simulink model "warplab_mimo_4x4"  (Simulink 6.6)
settings: Solver=ode45  StartTime=0.0  StopTime=50000  RelTol=1e-3
undefined symbols (not defined in the file): gcbh, xlBlockLoadCallback, xlGetSimulinkPeriod
libraries: xbsIndex_r4 x305, WARP_Blockset x16
(part 3 of 4)

== system warplab_mimo_4x4/Posedge ==
  D : Inport
  Delay : xbsIndex_r4/Delay  en=off  latency=1  dbl_ovrd=off  reg_retiming=off  block_type=delay
      settings: infoedit=Hardware notes: A delay line is a chain, each link of which is an SRL16 followed by a flip-flop. If register retiming is enabled, the delay line is a chain of flip-flops.  block_version=8.2
  Inverter : xbsIndex_r4/Inverter  en=off  latency=0  dbl_ovrd=off  block_type=inv
      settings: block_version=8.2
  Logical : xbsIndex_r4/Logical  logical_function=AND  inputs=2  en=off  latency=0  precision=Full  arith_type=Unsigned  n_bits=16  bin_pt=0  align_bp=on  dbl_ovrd=off  block_type=logical
      settings: block_version=8.2
  Q : Outport
  wires:
  D/1 -> Inverter/1, Logical/1
  Inverter/1 -> Delay/1
  Delay/1 -> Logical/2
  Logical/1 -> Q/1

== system warplab_mimo_4x4/Posedge1 ==
  D : Inport
  Delay : xbsIndex_r4/Delay  en=off  latency=1  dbl_ovrd=off  reg_retiming=off  block_type=delay
      settings: infoedit=Hardware notes: A delay line is a chain, each link of which is an SRL16 followed by a flip-flop. If register retiming is enabled, the delay line is a chain of flip-flops.  block_version=8.2
  Inverter : xbsIndex_r4/Inverter  en=off  latency=0  dbl_ovrd=off  block_type=inv
      settings: block_version=8.2
  Logical : xbsIndex_r4/Logical  logical_function=AND  inputs=2  en=off  latency=0  precision=Full  arith_type=Unsigned  n_bits=16  bin_pt=0  align_bp=on  dbl_ovrd=off  block_type=logical
      settings: block_version=8.2
  Q : Outport
  wires:
  Logical/1 -> Q/1
  Delay/1 -> Logical/2
  Inverter/1 -> Delay/1
  D/1 -> Logical/1, Inverter/1

== system warplab_mimo_4x4/Posedge2 ==
  D : Inport
  Delay : xbsIndex_r4/Delay  en=off  latency=1  dbl_ovrd=off  reg_retiming=off  block_type=delay
      settings: infoedit=Hardware notes: A delay line is a chain, each link of which is an SRL16 followed by a flip-flop. If register retiming is enabled, the delay line is a chain of flip-flops.  block_version=8.2
  Inverter : xbsIndex_r4/Inverter  en=off  latency=0  dbl_ovrd=off  block_type=inv
      settings: block_version=8.2
  Logical : xbsIndex_r4/Logical  logical_function=AND  inputs=2  en=off  latency=0  precision=Full  arith_type=Unsigned  n_bits=16  bin_pt=0  align_bp=on  dbl_ovrd=off  block_type=logical
      settings: block_version=8.2
  Q : Outport
  wires:
  Logical/1 -> Q/1
  Delay/1 -> Logical/2
  Inverter/1 -> Delay/1
  D/1 -> Logical/1, Inverter/1

== system warplab_mimo_4x4/Radio 1 Rx Buffers ==
  I/Q : Inport
  Addr : Inport  Port=2
  WE : Inport  Port=3
  EN : Inport  Port=4
  Convert1 : xbsIndex_r4/Convert  arith_type=Boolean  n_bits=16  bin_pt=14  quantization=Truncate  overflow=Wrap  latency=0  dbl_ovrd=off  pipeline=off  block_type=convert
      settings: block_version=8.2
  Gateway Out : xbsIndex_r4/Gateway Out  hdl_port=off  timing_constraint=None  locs_specified=off  LOCs={}  block_type=gatewayout
      settings: infoedit="Gateway out block.  Converts Xilinx fixed point inputs into ouputs of type Simulink integer, double, or fixed point.<P><P>Hardware notes:  In hardware these blocks become top level output ports or are discarded, depending on how they are configured."  block_version=10.1.2
  Gateway Out1 : xbsIndex_r4/Gateway Out  hdl_port=off  timing_constraint=None  locs_specified=off  LOCs={}  block_type=gatewayout
      settings: infoedit="Gateway out block.  Converts Xilinx fixed point inputs into ouputs of type Simulink integer, double, or fixed point.<P><P>Hardware notes:  In hardware these blocks become top level output ports or are discarded, depending on how they are configured."  block_version=10.1.2
  Logical : xbsIndex_r4/Logical  logical_function=AND  inputs=2  en=off  latency=0  precision=Full  arith_type=Unsigned  n_bits=16  bin_pt=0  align_bp=on  dbl_ovrd=off  block_type=logical
      settings: block_version=9.1.01
  Radio 1 I/Q Buffer : Subsystem
  Scope : Scope  NumInputPorts=2
      settings: YMin=-5~-5  YMax=5~5  SaveName=ScopeData2  MaxDataPoints=40000
  wires:
  Logical/1 -> Gateway Out1/1, Radio 1 I/Q Buffer/3(WE)
  Addr/1 -> Gateway Out/1, Radio 1 I/Q Buffer/1(Addr_14b)
  WE/1 -> Logical/1
  EN/1 -> Convert1/1
  Convert1/1 -> Logical/2
  I/Q/1 -> Radio 1 I/Q Buffer/2(I/Q_32b)
  Gateway Out/1 -> Scope/1
  Gateway Out1/1 -> Scope/2

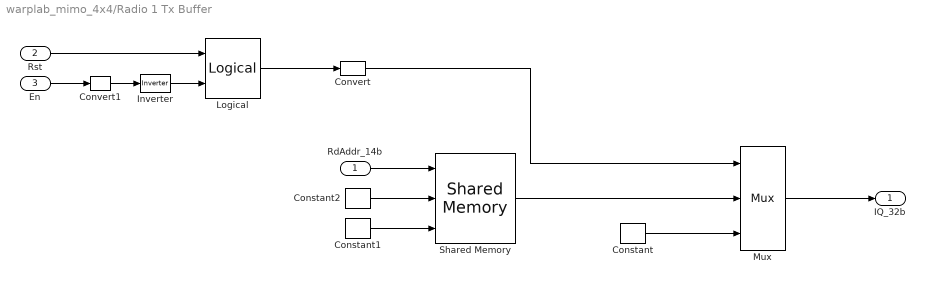
== system warplab_mimo_4x4/Radio 1 Tx Buffer ==
  RdAddr_14b : Inport
  Rst : Inport  Port=2
  En : Inport  Port=3
  Constant : xbsIndex_r4/Constant  arith_type=Unsigned  const=0  n_bits=32  bin_pt=0  explicit_period=off  period=1  equ=P=C  opselect=C  inp2=PCIN>>17  opr=+  inp1=P  carry=CIN  dbl_ovrd=off  block_type=constant
      settings: block_version=10.1.2
  Constant1 : xbsIndex_r4/Constant  arith_type=Boolean  const=0  n_bits=32  bin_pt=0  explicit_period=off  period=1  equ=P=C  opselect=C  inp2=PCIN>>17  opr=+  inp1=P  carry=CIN  dbl_ovrd=off  block_type=constant
      settings: block_version=10.1.2
  Constant2 : xbsIndex_r4/Constant  arith_type=Unsigned  const=0  n_bits=32  bin_pt=0  explicit_period=off  period=1  equ=P=C  opselect=C  inp2=PCIN>>17  opr=+  inp1=P  carry=CIN  dbl_ovrd=off  block_type=constant
      settings: block_version=10.1.2
  Convert : xbsIndex_r4/Convert  arith_type=Boolean  n_bits=16  bin_pt=14  quantization=Truncate  overflow=Wrap  latency=0  dbl_ovrd=off  pipeline=off  block_type=convert
      settings: block_version=8.2
  Convert1 : xbsIndex_r4/Convert  arith_type=Boolean  n_bits=16  bin_pt=14  quantization=Truncate  overflow=Wrap  latency=0  dbl_ovrd=off  pipeline=off  block_type=convert
      settings: block_version=8.2
  Inverter : xbsIndex_r4/Inverter  en=off  latency=0  dbl_ovrd=off  block_type=inv
      settings: block_version=9.1.01
  Logical : xbsIndex_r4/Logical  logical_function=OR  inputs=2  en=off  latency=0  precision=Full  arith_type=Unsigned  n_bits=16  bin_pt=0  align_bp=on  dbl_ovrd=off  block_type=logical
      settings: block_version=9.1.01
  Mux : xbsIndex_r4/Mux  inputs=2  en=off  latency=0  precision=Full  arith_type=Unsigned  n_bits=16  bin_pt=14  quantization=Truncate  overflow=Wrap  dbl_ovrd=off  block_type=mux
      settings: block_version=10.1.2
  Shared Memory : xbsIndex_r4/Shared Memory  shared_memory_name='TxBuff_Radio1'  depth=2^14  ownership=Locally Owned and Initialized  initVector=0  mutex=Unprotected  mode=Read and Write  write_mode=Read After Write  time_out=0  latency=1  explicit_data_type=on  arith_type=Unsigned  n_bits=32  bin_pt=0  implementation=Block RAM  use_rpm=off  block_type=shmem
      settings: AttributesFormatString=<< %<shared_memory_name> >>  block_version=10.1.2
  IQ_32b : Outport
  wires:
  Logical/1 -> Convert/1
  Convert/1 -> Mux/1
  Rst/1 -> Logical/1
  En/1 -> Convert1/1
  Convert1/1 -> Inverter/1
  Inverter/1 -> Logical/2
  RdAddr_14b/1 -> Shared Memory/1
  Constant/1 -> Mux/3
  Shared Memory/1 -> Mux/2
  Constant1/1 -> Shared Memory/3
  Constant2/1 -> Shared Memory/2
  Mux/1 -> IQ_32b/1

== system warplab_mimo_4x4/Radio 1 Inputs ==
  DebugRxBuffers : Inport
  ADC I : Subsystem
  ADC Q : Subsystem
  Concatenates_1 : Subsystem
  Gateway Out1 : xbsIndex_r4/Gateway Out  hdl_port=off  timing_constraint=None  locs_specified=off  LOCs={}  block_type=gatewayout
      settings: infoedit="Gateway out block.  Converts Xilinx fixed point inputs into ouputs of type Simulink integer, double, or fixed point.<P><P>Hardware notes:  In hardware these blocks become top level output ports or are discarded, depending on how they are configured."  block_version=10.1.2
  Gateway Out4 : xbsIndex_r4/Gateway Out  hdl_port=off  timing_constraint=None  locs_specified=off  LOCs={}  block_type=gatewayout
      settings: infoedit="Gateway out block.  Converts Xilinx fixed point inputs into ouputs of type Simulink integer, double, or fixed point.<P><P>Hardware notes:  In hardware these blocks become top level output ports or are discarded, depending on how they are configured."  block_version=10.1.2
  Scope : Scope  NumInputPorts=2
      settings: YMin=-5~-5  YMax=5~5
  Radio 1 I/Q : Outport
  wires:
  ADC Q/2(ADC Q) -> Concatenates_1/4(ADC_Q), Gateway Out1/1
  ADC Q/1(OTR Q) -> Concatenates_1/3(OTR_Q)
  ADC I/2(ADC I) -> Concatenates_1/2(ADC_I), Gateway Out4/1
  ADC I/1(OTR I) -> Concatenates_1/1(OTR_I)
  Concatenates_1/1(32b) -> Radio 1 I/Q/1
  Gateway Out4/1 -> Scope/1
  Gateway Out1/1 -> Scope/2
  DebugRxBuffers/1 -> ADC I/1(Debug), ADC Q/1(Debug)

== system warplab_mimo_4x4/Radio 1 Outputs ==
  32b : Inport
  16LSB : xbsIndex_r4/Slice  nbits=16  boolean_output=off  mode=Lower Bit Location + Width  bit1=0  base1=MSB of Input  bit0=0  base0=LSB of Input  dbl_ovrd=off  block_type=slice
      settings: infoedit="Extracts a given range of bits from each input sample and presents it at the output.  The output type is ordinarily unsigned with binary point at zero, but can be Boolean when the slice is one bit wide.<P><P>Hardware notes: In hardware this block costs nothing."  block_version=8.2
  16MSB : xbsIndex_r4/Slice  nbits=16  boolean_output=off  mode=Upper Bit Location + Width  bit1=0  base1=MSB of Input  bit0=0  base0=LSB of Input  dbl_ovrd=off  block_type=slice
      settings: infoedit="Extracts a given range of bits from each input sample and presents it at the output.  The output type is ordinarily unsigned with binary point at zero, but can be Boolean when the slice is one bit wide.<P><P>Hardware notes: In hardware this block costs nothing."  block_version=8.2
  Radio 1 DAC I : WARP_Blockset/WARP Radio Board ADC//DACs/Radio 1 DAC I  SystemSampleTime=-1
  Radio 1 DAC Q : WARP_Blockset/WARP Radio Board ADC//DACs/Radio 1 DAC Q  SystemSampleTime=-1
  Register : xbsIndex_r4/Register  init=0  rst=off  en=off  dbl_ovrd=off  block_type=register
      settings: block_version=8.2
  Register1 : xbsIndex_r4/Register  init=0  rst=off  en=off  dbl_ovrd=off  block_type=register
      settings: block_version=8.2
  Reinterpret : xbsIndex_r4/Reinterpret  force_arith_type=on  arith_type="Signed  (2's comp)"  force_bin_pt=on  bin_pt=15  block_type=reinterpret
      settings: infoedit="Changes signal type without altering the binary representation.   You can changed the signal between signed and unsigned, and relocate the binary point.<P><P>Hardware notes: In hardware this block costs nothing.<P><P>Example:  Suppose the input is 6 bits wide, signed, with 2 fractional bits, and the output is forced to unsigned with 0 fractional bits.  Then an input of -2.0 (1110.00 in binary 2's complement) becomes an output of 56 (111000 in binary)."  block_version=8.2
  Reinterpret1 : xbsIndex_r4/Reinterpret  force_arith_type=on  arith_type="Signed  (2's comp)"  force_bin_pt=on  bin_pt=15  block_type=reinterpret
      settings: infoedit="Changes signal type without altering the binary representation.   You can changed the signal between signed and unsigned, and relocate the binary point.<P><P>Hardware notes: In hardware this block costs nothing.<P><P>Example:  Suppose the input is 6 bits wide, signed, with 2 fractional bits, and the output is forced to unsigned with 0 fractional bits.  Then an input of -2.0 (1110.00 in binary 2's complement) becomes an output of 56 (111000 in binary)."  block_version=8.2
  Terminator1 : Terminator
  Terminator2 : Terminator
  wires:
  Radio 1 DAC Q/1 -> Terminator2/1
  Radio 1 DAC I/1 -> Terminator1/1
  Reinterpret1/1 -> Register1/1
  Reinterpret/1 -> Register/1
  16LSB/1 -> Reinterpret1/1
  16MSB/1 -> Reinterpret/1
  Register/1 -> Radio 1 DAC I/1
  Register1/1 -> Radio 1 DAC Q/1
  32b/1 -> 16MSB/1, 16LSB/1

== system warplab_mimo_4x4/Radio 2 Rx Buffers ==
  I/Q : Inport
  Addr : Inport  Port=2
  WE : Inport  Port=3
  EN : Inport  Port=4
  Convert1 : xbsIndex_r4/Convert  arith_type=Boolean  n_bits=16  bin_pt=14  quantization=Truncate  overflow=Wrap  latency=0  dbl_ovrd=off  pipeline=off  block_type=convert
      settings: block_version=8.2
  Gateway Out : xbsIndex_r4/Gateway Out  hdl_port=off  timing_constraint=None  locs_specified=off  LOCs={}  block_type=gatewayout
      settings: infoedit="Gateway out block.  Converts Xilinx fixed point inputs into ouputs of type Simulink integer, double, or fixed point.<P><P>Hardware notes:  In hardware these blocks become top level output ports or are discarded, depending on how they are configured."  block_version=10.1.2
  Gateway Out1 : xbsIndex_r4/Gateway Out  hdl_port=off  timing_constraint=None  locs_specified=off  LOCs={}  block_type=gatewayout
      settings: infoedit="Gateway out block.  Converts Xilinx fixed point inputs into ouputs of type Simulink integer, double, or fixed point.<P><P>Hardware notes:  In hardware these blocks become top level output ports or are discarded, depending on how they are configured."  block_version=10.1.2
  Logical : xbsIndex_r4/Logical  logical_function=AND  inputs=2  en=off  latency=0  precision=Full  arith_type=Unsigned  n_bits=16  bin_pt=0  align_bp=on  dbl_ovrd=off  block_type=logical
      settings: block_version=9.1.01
  Radio 2 I/Q Buffer : Subsystem
  Scope : Scope  NumInputPorts=2
      settings: YMin=-5~-5  YMax=5~5  SaveName=ScopeData2  MaxDataPoints=40000
  wires:
  Logical/1 -> Gateway Out1/1, Radio 2 I/Q Buffer/3(WE)
  Addr/1 -> Gateway Out/1, Radio 2 I/Q Buffer/1(Addr_14b)
  WE/1 -> Logical/1
  EN/1 -> Convert1/1
  Convert1/1 -> Logical/2
  I/Q/1 -> Radio 2 I/Q Buffer/2(I/Q_32b)
  Gateway Out/1 -> Scope/1
  Gateway Out1/1 -> Scope/2

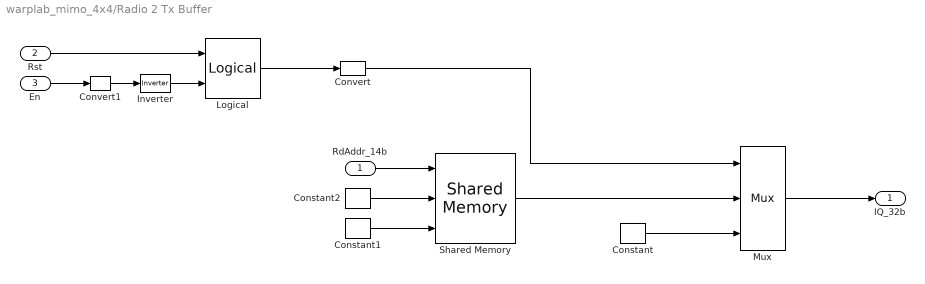
== system warplab_mimo_4x4/Radio 2 Tx Buffer ==
  RdAddr_14b : Inport
  Rst : Inport  Port=2
  En : Inport  Port=3
  Constant : xbsIndex_r4/Constant  arith_type=Unsigned  const=0  n_bits=32  bin_pt=0  explicit_period=off  period=1  equ=P=C  opselect=C  inp2=PCIN>>17  opr=+  inp1=P  carry=CIN  dbl_ovrd=off  block_type=constant
      settings: block_version=10.1.2
  Constant1 : xbsIndex_r4/Constant  arith_type=Boolean  const=0  n_bits=32  bin_pt=0  explicit_period=off  period=1  equ=P=C  opselect=C  inp2=PCIN>>17  opr=+  inp1=P  carry=CIN  dbl_ovrd=off  block_type=constant
      settings: block_version=10.1.2
  Constant2 : xbsIndex_r4/Constant  arith_type=Unsigned  const=0  n_bits=32  bin_pt=0  explicit_period=off  period=1  equ=P=C  opselect=C  inp2=PCIN>>17  opr=+  inp1=P  carry=CIN  dbl_ovrd=off  block_type=constant
      settings: block_version=10.1.2
  Convert : xbsIndex_r4/Convert  arith_type=Boolean  n_bits=16  bin_pt=14  quantization=Truncate  overflow=Wrap  latency=0  dbl_ovrd=off  pipeline=off  block_type=convert
      settings: block_version=8.2
  Convert1 : xbsIndex_r4/Convert  arith_type=Boolean  n_bits=16  bin_pt=14  quantization=Truncate  overflow=Wrap  latency=0  dbl_ovrd=off  pipeline=off  block_type=convert
      settings: block_version=8.2
  Inverter : xbsIndex_r4/Inverter  en=off  latency=0  dbl_ovrd=off  block_type=inv
      settings: block_version=9.1.01
  Logical : xbsIndex_r4/Logical  logical_function=OR  inputs=2  en=off  latency=0  precision=Full  arith_type=Unsigned  n_bits=16  bin_pt=0  align_bp=on  dbl_ovrd=off  block_type=logical
      settings: block_version=9.1.01
  Mux : xbsIndex_r4/Mux  inputs=2  en=off  latency=0  precision=Full  arith_type=Unsigned  n_bits=16  bin_pt=14  quantization=Truncate  overflow=Wrap  dbl_ovrd=off  block_type=mux
      settings: block_version=10.1.2
  Shared Memory : xbsIndex_r4/Shared Memory  shared_memory_name='TxBuff_Radio2'  depth=2^14  ownership=Locally Owned and Initialized  initVector=0  mutex=Unprotected  mode=Read and Write  write_mode=Read After Write  time_out=0  latency=1  explicit_data_type=on  arith_type=Unsigned  n_bits=32  bin_pt=0  implementation=Block RAM  use_rpm=off  block_type=shmem
      settings: AttributesFormatString=<< %<shared_memory_name> >>  block_version=10.1.2
  IQ_32b : Outport
  wires:
  Logical/1 -> Convert/1
  Convert/1 -> Mux/1
  Rst/1 -> Logical/1
  En/1 -> Convert1/1
  Convert1/1 -> Inverter/1
  Inverter/1 -> Logical/2
  RdAddr_14b/1 -> Shared Memory/1
  Constant/1 -> Mux/3
  Shared Memory/1 -> Mux/2
  Constant1/1 -> Shared Memory/3
  Constant2/1 -> Shared Memory/2
  Mux/1 -> IQ_32b/1

== system warplab_mimo_4x4/Radio 2 Inputs ==
  DebugRxBuffers : Inport
  ADC I : Subsystem
  ADC Q : Subsystem
  Concatenates_1 : Subsystem
  Gateway Out1 : xbsIndex_r4/Gateway Out  hdl_port=off  timing_constraint=None  locs_specified=off  LOCs={}  block_type=gatewayout
      settings: infoedit="Gateway out block.  Converts Xilinx fixed point inputs into ouputs of type Simulink integer, double, or fixed point.<P><P>Hardware notes:  In hardware these blocks become top level output ports or are discarded, depending on how they are configured."  block_version=10.1.2
  Gateway Out4 : xbsIndex_r4/Gateway Out  hdl_port=off  timing_constraint=None  locs_specified=off  LOCs={}  block_type=gatewayout
      settings: infoedit="Gateway out block.  Converts Xilinx fixed point inputs into ouputs of type Simulink integer, double, or fixed point.<P><P>Hardware notes:  In hardware these blocks become top level output ports or are discarded, depending on how they are configured."  block_version=10.1.2
  Scope : Scope  NumInputPorts=2
      settings: YMin=-5~-5  YMax=5~5
  Radio 2 I/Q : Outport
  wires:
  ADC Q/2(ADC Q) -> Concatenates_1/4(ADC_Q), Gateway Out1/1
  ADC Q/1(OTR Q) -> Concatenates_1/3(OTR_Q)
  ADC I/2(ADC I) -> Concatenates_1/2(ADC_I), Gateway Out4/1
  ADC I/1(OTR I) -> Concatenates_1/1(OTR_I)
  Concatenates_1/1(32b) -> Radio 2 I/Q/1
  Gateway Out4/1 -> Scope/1
  Gateway Out1/1 -> Scope/2
  DebugRxBuffers/1 -> ADC I/1(Debug), ADC Q/1(Debug)

== system warplab_mimo_4x4/Radio 2 Outputs ==
  32b : Inport
  16LSB : xbsIndex_r4/Slice  nbits=16  boolean_output=off  mode=Lower Bit Location + Width  bit1=0  base1=MSB of Input  bit0=0  base0=LSB of Input  dbl_ovrd=off  block_type=slice
      settings: infoedit="Extracts a given range of bits from each input sample and presents it at the output.  The output type is ordinarily unsigned with binary point at zero, but can be Boolean when the slice is one bit wide.<P><P>Hardware notes: In hardware this block costs nothing."  block_version=8.2
  16MSB : xbsIndex_r4/Slice  nbits=16  boolean_output=off  mode=Upper Bit Location + Width  bit1=0  base1=MSB of Input  bit0=0  base0=LSB of Input  dbl_ovrd=off  block_type=slice
      settings: infoedit="Extracts a given range of bits from each input sample and presents it at the output.  The output type is ordinarily unsigned with binary point at zero, but can be Boolean when the slice is one bit wide.<P><P>Hardware notes: In hardware this block costs nothing."  block_version=8.2
  Radio 2 DAC I : WARP_Blockset/WARP Radio Board ADC//DACs/Radio 2 DAC I  SystemSampleTime=-1
  Radio 2 DAC Q : WARP_Blockset/WARP Radio Board ADC//DACs/Radio 2 DAC Q  SystemSampleTime=-1
  Register : xbsIndex_r4/Register  init=0  rst=off  en=off  dbl_ovrd=off  block_type=register
      settings: block_version=8.2
  Register1 : xbsIndex_r4/Register  init=0  rst=off  en=off  dbl_ovrd=off  block_type=register
      settings: block_version=8.2
  Reinterpret : xbsIndex_r4/Reinterpret  force_arith_type=on  arith_type="Signed  (2's comp)"  force_bin_pt=on  bin_pt=15  block_type=reinterpret
      settings: infoedit="Changes signal type without altering the binary representation.   You can changed the signal between signed and unsigned, and relocate the binary point.<P><P>Hardware notes: In hardware this block costs nothing.<P><P>Example:  Suppose the input is 6 bits wide, signed, with 2 fractional bits, and the output is forced to unsigned with 0 fractional bits.  Then an input of -2.0 (1110.00 in binary 2's complement) becomes an output of 56 (111000 in binary)."  block_version=8.2
  Reinterpret1 : xbsIndex_r4/Reinterpret  force_arith_type=on  arith_type="Signed  (2's comp)"  force_bin_pt=on  bin_pt=15  block_type=reinterpret
      settings: infoedit="Changes signal type without altering the binary representation.   You can changed the signal between signed and unsigned, and relocate the binary point.<P><P>Hardware notes: In hardware this block costs nothing.<P><P>Example:  Suppose the input is 6 bits wide, signed, with 2 fractional bits, and the output is forced to unsigned with 0 fractional bits.  Then an input of -2.0 (1110.00 in binary 2's complement) becomes an output of 56 (111000 in binary)."  block_version=8.2
  Terminator1 : Terminator
  Terminator2 : Terminator
  wires:
  Radio 2 DAC Q/1 -> Terminator2/1
  Radio 2 DAC I/1 -> Terminator1/1
  Reinterpret1/1 -> Register1/1
  Reinterpret/1 -> Register/1
  16LSB/1 -> Reinterpret1/1
  16MSB/1 -> Reinterpret/1
  Register/1 -> Radio 2 DAC I/1
  Register1/1 -> Radio 2 DAC Q/1
  32b/1 -> 16MSB/1, 16LSB/1

== system warplab_mimo_4x4/Radio 3 Rx Buffers ==
  I/Q : Inport
  Addr : Inport  Port=2
  WE : Inport  Port=3
  EN : Inport  Port=4
  Convert1 : xbsIndex_r4/Convert  arith_type=Boolean  n_bits=16  bin_pt=14  quantization=Truncate  overflow=Wrap  latency=0  dbl_ovrd=off  pipeline=off  block_type=convert
      settings: block_version=8.2
  Gateway Out : xbsIndex_r4/Gateway Out  hdl_port=off  timing_constraint=None  locs_specified=off  LOCs={}  block_type=gatewayout
      settings: infoedit="Gateway out block.  Converts Xilinx fixed point inputs into ouputs of type Simulink integer, double, or fixed point.<P><P>Hardware notes:  In hardware these blocks become top level output ports or are discarded, depending on how they are configured."  block_version=10.1.2
  Gateway Out1 : xbsIndex_r4/Gateway Out  hdl_port=off  timing_constraint=None  locs_specified=off  LOCs={}  block_type=gatewayout
      settings: infoedit="Gateway out block.  Converts Xilinx fixed point inputs into ouputs of type Simulink integer, double, or fixed point.<P><P>Hardware notes:  In hardware these blocks become top level output ports or are discarded, depending on how they are configured."  block_version=10.1.2
  Logical : xbsIndex_r4/Logical  logical_function=AND  inputs=2  en=off  latency=0  precision=Full  arith_type=Unsigned  n_bits=16  bin_pt=0  align_bp=on  dbl_ovrd=off  block_type=logical
      settings: block_version=9.1.01
  Radio 3 I/Q Buffer : Subsystem
  Scope : Scope  NumInputPorts=2
      settings: YMin=-5~-5  YMax=5~5  SaveName=ScopeData2  MaxDataPoints=40000
  wires:
  Gateway Out1/1 -> Scope/2
  Gateway Out/1 -> Scope/1
  I/Q/1 -> Radio 3 I/Q Buffer/2(I/Q_32b)
  Convert1/1 -> Logical/2
  EN/1 -> Convert1/1
  WE/1 -> Logical/1
  Addr/1 -> Gateway Out/1, Radio 3 I/Q Buffer/1(Addr_14b)
  Logical/1 -> Gateway Out1/1, Radio 3 I/Q Buffer/3(WE)

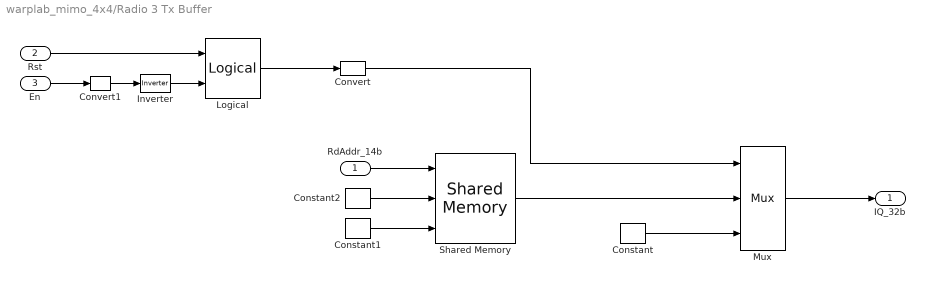
== system warplab_mimo_4x4/Radio 3 Tx Buffer ==
  RdAddr_14b : Inport
  Rst : Inport  Port=2
  En : Inport  Port=3
  Constant : xbsIndex_r4/Constant  arith_type=Unsigned  const=0  n_bits=32  bin_pt=0  explicit_period=off  period=1  equ=P=C  opselect=C  inp2=PCIN>>17  opr=+  inp1=P  carry=CIN  dbl_ovrd=off  block_type=constant
      settings: block_version=10.1.2
  Constant1 : xbsIndex_r4/Constant  arith_type=Boolean  const=0  n_bits=32  bin_pt=0  explicit_period=off  period=1  equ=P=C  opselect=C  inp2=PCIN>>17  opr=+  inp1=P  carry=CIN  dbl_ovrd=off  block_type=constant
      settings: block_version=10.1.2
  Constant2 : xbsIndex_r4/Constant  arith_type=Unsigned  const=0  n_bits=32  bin_pt=0  explicit_period=off  period=1  equ=P=C  opselect=C  inp2=PCIN>>17  opr=+  inp1=P  carry=CIN  dbl_ovrd=off  block_type=constant
      settings: block_version=10.1.2
  Convert : xbsIndex_r4/Convert  arith_type=Boolean  n_bits=16  bin_pt=14  quantization=Truncate  overflow=Wrap  latency=0  dbl_ovrd=off  pipeline=off  block_type=convert
      settings: block_version=8.2
  Convert1 : xbsIndex_r4/Convert  arith_type=Boolean  n_bits=16  bin_pt=14  quantization=Truncate  overflow=Wrap  latency=0  dbl_ovrd=off  pipeline=off  block_type=convert
      settings: block_version=8.2
  Inverter : xbsIndex_r4/Inverter  en=off  latency=0  dbl_ovrd=off  block_type=inv
      settings: block_version=9.1.01
  Logical : xbsIndex_r4/Logical  logical_function=OR  inputs=2  en=off  latency=0  precision=Full  arith_type=Unsigned  n_bits=16  bin_pt=0  align_bp=on  dbl_ovrd=off  block_type=logical
      settings: block_version=9.1.01
  Mux : xbsIndex_r4/Mux  inputs=2  en=off  latency=0  precision=Full  arith_type=Unsigned  n_bits=16  bin_pt=14  quantization=Truncate  overflow=Wrap  dbl_ovrd=off  block_type=mux
      settings: block_version=10.1.2
  Shared Memory : xbsIndex_r4/Shared Memory  shared_memory_name='TxBuff_Radio3'  depth=2^14  ownership=Locally Owned and Initialized  initVector=0  mutex=Unprotected  mode=Read and Write  write_mode=Read After Write  time_out=0  latency=1  explicit_data_type=on  arith_type=Unsigned  n_bits=32  bin_pt=0  implementation=Block RAM  use_rpm=off  block_type=shmem
      settings: AttributesFormatString=<< %<shared_memory_name> >>  block_version=10.1.2
  IQ_32b : Outport
  wires:
  Mux/1 -> IQ_32b/1
  Constant2/1 -> Shared Memory/2
  Constant1/1 -> Shared Memory/3
  Shared Memory/1 -> Mux/2
  Constant/1 -> Mux/3
  RdAddr_14b/1 -> Shared Memory/1
  Inverter/1 -> Logical/2
  Convert1/1 -> Inverter/1
  En/1 -> Convert1/1
  Rst/1 -> Logical/1
  Convert/1 -> Mux/1
  Logical/1 -> Convert/1

== system warplab_mimo_4x4/Radio 3 Inputs ==
  DebugRxBuffers : Inport
  ADC I : Subsystem
  ADC Q : Subsystem
  Concatenates_1 : Subsystem
  Gateway Out1 : xbsIndex_r4/Gateway Out  hdl_port=off  timing_constraint=None  locs_specified=off  LOCs={}  block_type=gatewayout
      settings: infoedit="Gateway out block.  Converts Xilinx fixed point inputs into ouputs of type Simulink integer, double, or fixed point.<P><P>Hardware notes:  In hardware these blocks become top level output ports or are discarded, depending on how they are configured."  block_version=10.1.2
  Gateway Out4 : xbsIndex_r4/Gateway Out  hdl_port=off  timing_constraint=None  locs_specified=off  LOCs={}  block_type=gatewayout
      settings: infoedit="Gateway out block.  Converts Xilinx fixed point inputs into ouputs of type Simulink integer, double, or fixed point.<P><P>Hardware notes:  In hardware these blocks become top level output ports or are discarded, depending on how they are configured."  block_version=10.1.2
  Scope : Scope  NumInputPorts=2
      settings: YMin=-5~-5  YMax=5~5
  Radio 3 I/Q : Outport
  wires:
  ADC Q/2(ADC Q) -> Concatenates_1/4(ADC_Q), Gateway Out1/1
  ADC Q/1(OTR Q) -> Concatenates_1/3(OTR_Q)
  ADC I/2(ADC I) -> Concatenates_1/2(ADC_I), Gateway Out4/1
  ADC I/1(OTR I) -> Concatenates_1/1(OTR_I)
  Concatenates_1/1(32b) -> Radio 3 I/Q/1
  Gateway Out4/1 -> Scope/1
  Gateway Out1/1 -> Scope/2
  DebugRxBuffers/1 -> ADC I/1(Debug), ADC Q/1(Debug)

== system warplab_mimo_4x4/Radio 3 Outputs ==
  32b : Inport
  16LSB : xbsIndex_r4/Slice  nbits=16  boolean_output=off  mode=Lower Bit Location + Width  bit1=0  base1=MSB of Input  bit0=0  base0=LSB of Input  dbl_ovrd=off  block_type=slice
      settings: infoedit="Extracts a given range of bits from each input sample and presents it at the output.  The output type is ordinarily unsigned with binary point at zero, but can be Boolean when the slice is one bit wide.<P><P>Hardware notes: In hardware this block costs nothing."  block_version=9.1.01
  16MSB : xbsIndex_r4/Slice  nbits=16  boolean_output=off  mode=Upper Bit Location + Width  bit1=0  base1=MSB of Input  bit0=0  base0=LSB of Input  dbl_ovrd=off  block_type=slice
      settings: infoedit="Extracts a given range of bits from each input sample and presents it at the output.  The output type is ordinarily unsigned with binary point at zero, but can be Boolean when the slice is one bit wide.<P><P>Hardware notes: In hardware this block costs nothing."  block_version=9.1.01
  Radio 3 DAC I : WARP_Blockset/WARP Radio Board ADC//DACs/Radio 3 DAC I  SystemSampleTime=-1
  Radio 3 DAC Q : WARP_Blockset/WARP Radio Board ADC//DACs/Radio 3 DAC Q  SystemSampleTime=-1
  Register : xbsIndex_r4/Register  init=0  rst=off  en=off  dbl_ovrd=off  block_type=register
      settings: block_version=9.1.01
  Register1 : xbsIndex_r4/Register  init=0  rst=off  en=off  dbl_ovrd=off  block_type=register
      settings: block_version=9.1.01
  Reinterpret : xbsIndex_r4/Reinterpret  force_arith_type=on  arith_type="Signed  (2's comp)"  force_bin_pt=on  bin_pt=15  block_type=reinterpret
      settings: infoedit="Changes signal type without altering the binary representation.   You can changed the signal between signed and unsigned, and relocate the binary point.<P><P>Hardware notes: In hardware this block costs nothing.<P><P>Example:  Suppose the input is 6 bits wide, signed, with 2 fractional bits, and the output is forced to unsigned with 0 fractional bits.  Then an input of -2.0 (1110.00 in binary 2's complement) becomes an output of 56 (111000 in binary)."  block_version=9.1.01
  Reinterpret1 : xbsIndex_r4/Reinterpret  force_arith_type=on  arith_type="Signed  (2's comp)"  force_bin_pt=on  bin_pt=15  block_type=reinterpret
      settings: infoedit="Changes signal type without altering the binary representation.   You can changed the signal between signed and unsigned, and relocate the binary point.<P><P>Hardware notes: In hardware this block costs nothing.<P><P>Example:  Suppose the input is 6 bits wide, signed, with 2 fractional bits, and the output is forced to unsigned with 0 fractional bits.  Then an input of -2.0 (1110.00 in binary 2's complement) becomes an output of 56 (111000 in binary)."  block_version=9.1.01
  Terminator : Terminator
  Terminator1 : Terminator
  wires:
  32b/1 -> 16LSB/1, 16MSB/1
  16MSB/1 -> Reinterpret/1
  16LSB/1 -> Reinterpret1/1
  Reinterpret/1 -> Register/1
  Reinterpret1/1 -> Register1/1
  Register/1 -> Radio 3 DAC I/1
  Register1/1 -> Radio 3 DAC Q/1
  Radio 3 DAC I/1 -> Terminator/1
  Radio 3 DAC Q/1 -> Terminator1/1

== system warplab_mimo_4x4/Radio 4 Rx Buffers ==
  I/Q : Inport
  Addr : Inport  Port=2
  WE : Inport  Port=3
  EN : Inport  Port=4
  Convert1 : xbsIndex_r4/Convert  arith_type=Boolean  n_bits=16  bin_pt=14  quantization=Truncate  overflow=Wrap  latency=0  dbl_ovrd=off  pipeline=off  block_type=convert
      settings: block_version=8.2
  Gateway Out : xbsIndex_r4/Gateway Out  hdl_port=off  timing_constraint=None  locs_specified=off  LOCs={}  block_type=gatewayout
      settings: infoedit="Gateway out block.  Converts Xilinx fixed point inputs into ouputs of type Simulink integer, double, or fixed point.<P><P>Hardware notes:  In hardware these blocks become top level output ports or are discarded, depending on how they are configured."  block_version=10.1.2
  Gateway Out1 : xbsIndex_r4/Gateway Out  hdl_port=off  timing_constraint=None  locs_specified=off  LOCs={}  block_type=gatewayout
      settings: infoedit="Gateway out block.  Converts Xilinx fixed point inputs into ouputs of type Simulink integer, double, or fixed point.<P><P>Hardware notes:  In hardware these blocks become top level output ports or are discarded, depending on how they are configured."  block_version=10.1.2
  Logical : xbsIndex_r4/Logical  logical_function=AND  inputs=2  en=off  latency=0  precision=Full  arith_type=Unsigned  n_bits=16  bin_pt=0  align_bp=on  dbl_ovrd=off  block_type=logical
      settings: block_version=9.1.01
  Radio 4 I/Q Buffer : Subsystem
  Scope : Scope  NumInputPorts=2
      settings: YMin=-5~-5  YMax=5~5  SaveName=ScopeData2  MaxDataPoints=40000
  wires:
  Gateway Out1/1 -> Scope/2
  Gateway Out/1 -> Scope/1
  I/Q/1 -> Radio 4 I/Q Buffer/2(I/Q_32b)
  Convert1/1 -> Logical/2
  EN/1 -> Convert1/1
  WE/1 -> Logical/1
  Addr/1 -> Gateway Out/1, Radio 4 I/Q Buffer/1(Addr_14b)
  Logical/1 -> Gateway Out1/1, Radio 4 I/Q Buffer/3(WE)

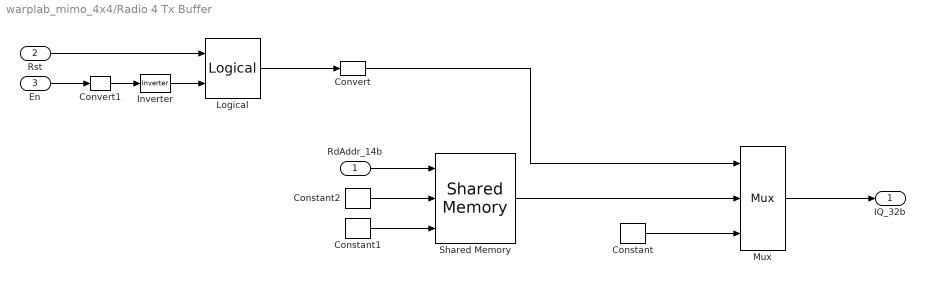
== system warplab_mimo_4x4/Radio 4 Tx Buffer ==
  RdAddr_14b : Inport
  Rst : Inport  Port=2
  En : Inport  Port=3
  Constant : xbsIndex_r4/Constant  arith_type=Unsigned  const=0  n_bits=32  bin_pt=0  explicit_period=off  period=1  equ=P=C  opselect=C  inp2=PCIN>>17  opr=+  inp1=P  carry=CIN  dbl_ovrd=off  block_type=constant
      settings: block_version=10.1.2
  Constant1 : xbsIndex_r4/Constant  arith_type=Boolean  const=0  n_bits=32  bin_pt=0  explicit_period=off  period=1  equ=P=C  opselect=C  inp2=PCIN>>17  opr=+  inp1=P  carry=CIN  dbl_ovrd=off  block_type=constant
      settings: block_version=10.1.2
  Constant2 : xbsIndex_r4/Constant  arith_type=Unsigned  const=0  n_bits=32  bin_pt=0  explicit_period=off  period=1  equ=P=C  opselect=C  inp2=PCIN>>17  opr=+  inp1=P  carry=CIN  dbl_ovrd=off  block_type=constant
      settings: block_version=10.1.2
  Convert : xbsIndex_r4/Convert  arith_type=Boolean  n_bits=16  bin_pt=14  quantization=Truncate  overflow=Wrap  latency=0  dbl_ovrd=off  pipeline=off  block_type=convert
      settings: block_version=8.2
  Convert1 : xbsIndex_r4/Convert  arith_type=Boolean  n_bits=16  bin_pt=14  quantization=Truncate  overflow=Wrap  latency=0  dbl_ovrd=off  pipeline=off  block_type=convert
      settings: block_version=8.2
  Inverter : xbsIndex_r4/Inverter  en=off  latency=0  dbl_ovrd=off  block_type=inv
      settings: block_version=9.1.01
  Logical : xbsIndex_r4/Logical  logical_function=OR  inputs=2  en=off  latency=0  precision=Full  arith_type=Unsigned  n_bits=16  bin_pt=0  align_bp=on  dbl_ovrd=off  block_type=logical
      settings: block_version=9.1.01
  Mux : xbsIndex_r4/Mux  inputs=2  en=off  latency=0  precision=Full  arith_type=Unsigned  n_bits=16  bin_pt=14  quantization=Truncate  overflow=Wrap  dbl_ovrd=off  block_type=mux
      settings: block_version=10.1.2
  Shared Memory : xbsIndex_r4/Shared Memory  shared_memory_name='TxBuff_Radio4'  depth=2^14  ownership=Locally Owned and Initialized  initVector=0  mutex=Unprotected  mode=Read and Write  write_mode=Read After Write  time_out=0  latency=1  explicit_data_type=on  arith_type=Unsigned  n_bits=32  bin_pt=0  implementation=Block RAM  use_rpm=off  block_type=shmem
      settings: AttributesFormatString=<< %<shared_memory_name> >>  block_version=10.1.2
  IQ_32b : Outport
  wires:
  Mux/1 -> IQ_32b/1
  Constant2/1 -> Shared Memory/2
  Constant1/1 -> Shared Memory/3
  Shared Memory/1 -> Mux/2
  Constant/1 -> Mux/3
  RdAddr_14b/1 -> Shared Memory/1
  Inverter/1 -> Logical/2
  Convert1/1 -> Inverter/1
  En/1 -> Convert1/1
  Rst/1 -> Logical/1
  Convert/1 -> Mux/1
  Logical/1 -> Convert/1

== system warplab_mimo_4x4/Radio 4 Inputs ==
  DebugRxBuffers : Inport
  ADC I : Subsystem
  ADC Q : Subsystem
  Concatenates_1 : Subsystem
  Gateway Out1 : xbsIndex_r4/Gateway Out  hdl_port=off  timing_constraint=None  locs_specified=off  LOCs={}  block_type=gatewayout
      settings: infoedit="Gateway out block.  Converts Xilinx fixed point inputs into ouputs of type Simulink integer, double, or fixed point.<P><P>Hardware notes:  In hardware these blocks become top level output ports or are discarded, depending on how they are configured."  block_version=10.1.2
  Gateway Out4 : xbsIndex_r4/Gateway Out  hdl_port=off  timing_constraint=None  locs_specified=off  LOCs={}  block_type=gatewayout
      settings: infoedit="Gateway out block.  Converts Xilinx fixed point inputs into ouputs of type Simulink integer, double, or fixed point.<P><P>Hardware notes:  In hardware these blocks become top level output ports or are discarded, depending on how they are configured."  block_version=10.1.2
  Scope : Scope  NumInputPorts=2
      settings: YMin=-5~-5  YMax=5~5
  Radio 4 I/Q : Outport
  wires:
  ADC Q/2(ADC Q) -> Concatenates_1/4(ADC_Q), Gateway Out1/1
  ADC Q/1(OTR Q) -> Concatenates_1/3(OTR_Q)
  ADC I/2(ADC I) -> Concatenates_1/2(ADC_I), Gateway Out4/1
  ADC I/1(OTR I) -> Concatenates_1/1(OTR_I)
  Concatenates_1/1(32b) -> Radio 4 I/Q/1
  Gateway Out4/1 -> Scope/1
  Gateway Out1/1 -> Scope/2
  DebugRxBuffers/1 -> ADC I/1(Debug), ADC Q/1(Debug)

== system warplab_mimo_4x4/Radio 4 Outputs ==
  32b : Inport
  16LSB : xbsIndex_r4/Slice  nbits=16  boolean_output=off  mode=Lower Bit Location + Width  bit1=0  base1=MSB of Input  bit0=0  base0=LSB of Input  dbl_ovrd=off  block_type=slice
      settings: infoedit="Extracts a given range of bits from each input sample and presents it at the output.  The output type is ordinarily unsigned with binary point at zero, but can be Boolean when the slice is one bit wide.<P><P>Hardware notes: In hardware this block costs nothing."  block_version=9.1.01
  16MSB : xbsIndex_r4/Slice  nbits=16  boolean_output=off  mode=Upper Bit Location + Width  bit1=0  base1=MSB of Input  bit0=0  base0=LSB of Input  dbl_ovrd=off  block_type=slice
      settings: infoedit="Extracts a given range of bits from each input sample and presents it at the output.  The output type is ordinarily unsigned with binary point at zero, but can be Boolean when the slice is one bit wide.<P><P>Hardware notes: In hardware this block costs nothing."  block_version=9.1.01
  Radio 4 DAC I : WARP_Blockset/WARP Radio Board ADC//DACs/Radio 4 DAC I  SystemSampleTime=-1
  Radio 4 DAC Q : WARP_Blockset/WARP Radio Board ADC//DACs/Radio 4 DAC Q  SystemSampleTime=-1
  Register : xbsIndex_r4/Register  init=0  rst=off  en=off  dbl_ovrd=off  block_type=register
      settings: block_version=9.1.01
  Register1 : xbsIndex_r4/Register  init=0  rst=off  en=off  dbl_ovrd=off  block_type=register
      settings: block_version=9.1.01
  Reinterpret : xbsIndex_r4/Reinterpret  force_arith_type=on  arith_type="Signed  (2's comp)"  force_bin_pt=on  bin_pt=15  block_type=reinterpret
      settings: infoedit="Changes signal type without altering the binary representation.   You can changed the signal between signed and unsigned, and relocate the binary point.<P><P>Hardware notes: In hardware this block costs nothing.<P><P>Example:  Suppose the input is 6 bits wide, signed, with 2 fractional bits, and the output is forced to unsigned with 0 fractional bits.  Then an input of -2.0 (1110.00 in binary 2's complement) becomes an output of 56 (111000 in binary)."  block_version=9.1.01
  Reinterpret1 : xbsIndex_r4/Reinterpret  force_arith_type=on  arith_type="Signed  (2's comp)"  force_bin_pt=on  bin_pt=15  block_type=reinterpret
      settings: infoedit="Changes signal type without altering the binary representation.   You can changed the signal between signed and unsigned, and relocate the binary point.<P><P>Hardware notes: In hardware this block costs nothing.<P><P>Example:  Suppose the input is 6 bits wide, signed, with 2 fractional bits, and the output is forced to unsigned with 0 fractional bits.  Then an input of -2.0 (1110.00 in binary 2's complement) becomes an output of 56 (111000 in binary)."  block_version=9.1.01
  Terminator : Terminator
  Terminator1 : Terminator
  wires:
  32b/1 -> 16LSB/1, 16MSB/1
  16MSB/1 -> Reinterpret/1
  16LSB/1 -> Reinterpret1/1
  Reinterpret/1 -> Register/1
  Reinterpret1/1 -> Register1/1
  Register/1 -> Radio 4 DAC I/1
  Register1/1 -> Radio 4 DAC Q/1
  Radio 4 DAC I/1 -> Terminator/1
  Radio 4 DAC Q/1 -> Terminator1/1

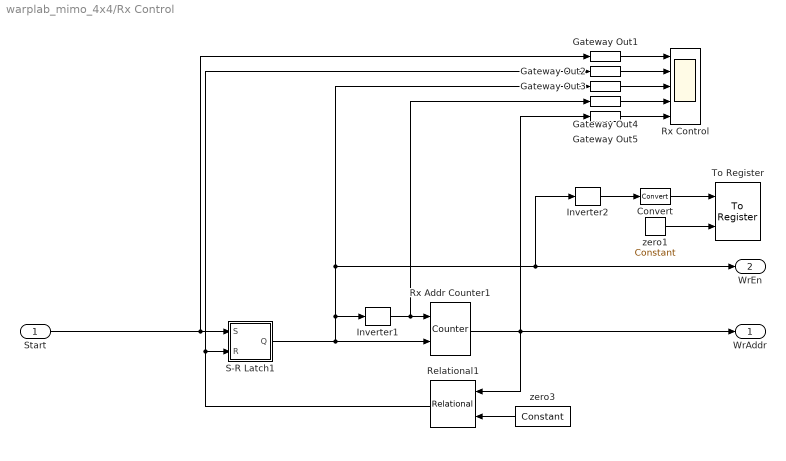
== system warplab_mimo_4x4/Rx Control ==
  Start : Inport
  Convert : xbsIndex_r4/Convert  arith_type=Unsigned  n_bits=1  bin_pt=0  quantization=Truncate  overflow=Wrap  latency=0  dbl_ovrd=off  pipeline=off  block_type=convert
      settings: block_version=10.1.2
  Gateway Out{1..5} (5 alike) : xbsIndex_r4/Gateway Out  hdl_port=off  timing_constraint=None  locs_specified=off  LOCs={}  block_type=gatewayout
      settings: infoedit="Gateway out block.  Converts Xilinx fixed point inputs into ouputs of type Simulink integer, double, or fixed point.<P><P>Hardware notes:  In hardware these blocks become top level output ports or are discarded, depending on how they are configured."  block_version=10.1.2
  Inverter1 : xbsIndex_r4/Inverter  en=off  latency=0  dbl_ovrd=off  block_type=inv
      settings: block_version=8.2
  Inverter2 : xbsIndex_r4/Inverter  en=off  latency=0  dbl_ovrd=off  block_type=inv
      settings: block_version=8.2
  Relational1 : xbsIndex_r4/Relational  Orientation=left  mode=a>=b  en=off  latency=0  dbl_ovrd=off  block_type=relational
      settings: block_version=8.2
  Rx Addr Counter1 : xbsIndex_r4/Counter  cnt_type=Free Running  cnt_to=Inf  operation=Up  start_count=0  cnt_by_val=1  arith_type=Unsigned  n_bits=14  bin_pt=0  load_pin=off  rst=on  en=on  explicit_period=off  period=1  dbl_ovrd=off  use_behavioral_HDL=off  use_rpm=off  implementation=Fabric  block_type=counter
      settings: block_version=8.2
  Rx Control : Scope  NumInputPorts=5
      settings: TimeRange=70000  YMin=0~0~0~0~0  YMax=1~1~1~1~20000
  S-R Latch1 : Subsystem
  To Register : xbsIndex_r4/To Register  shared_memory_name='CaptureDone'  init=0  ownership=Locally owned and initialized  explicit_data_type=on  arith_type=Unsigned  n_bits=1  bin_pt=0  dbl_ovrd=off  block_type=toreg
      settings: AttributesFormatString=CaptureDone\n<< %<shared_memory_name> >>  infoedit="Register block that writes data to a shared memory register.  Delay of one sample period."  block_version=8.2
  zero1 : xbsIndex_r4/Constant  arith_type=Boolean  const=1  n_bits=1  bin_pt=0  explicit_period=off  period=1  equ=P=C  opselect=C  inp2=PCIN>>17  opr=+  inp1=P  carry=CIN  dbl_ovrd=off  block_type=constant
      settings: block_version=VER_STRING_GOES_HERE
  zero3 : xbsIndex_r4/Constant  Orientation=left  arith_type=Unsigned  const=2^14-1  n_bits=14  bin_pt=0  explicit_period=off  period=1  equ=P=C  opselect=C  inp2=PCIN>>17  opr=+  inp1=P  carry=CIN  dbl_ovrd=off  block_type=constant
      settings: block_version=VER_STRING_GOES_HERE
  WrAddr : Outport
  WrEn : Outport  Port=2
  wires:
  Start/1 -> S-R Latch1/1(S), Gateway Out1/1
  S-R Latch1/1(Q) -> Rx Addr Counter1/2, Inverter1/1, WrEn/1, Inverter2/1, Gateway Out3/1
  Inverter1/1 -> Rx Addr Counter1/1, Gateway Out4/1
  Rx Addr Counter1/1 -> Relational1/1, WrAddr/1, Gateway Out5/1
  Gateway Out5/1 -> Rx Control/5
  Gateway Out4/1 -> Rx Control/4
  Gateway Out3/1 -> Rx Control/3
  Gateway Out2/1 -> Rx Control/2
  Gateway Out1/1 -> Rx Control/1
  zero3/1 -> Relational1/2
  Relational1/1 -> S-R Latch1/2(R), Gateway Out2/1
  zero1/1 -> To Register/2
  Inverter2/1 -> Convert/1
  Convert/1 -> To Register/1

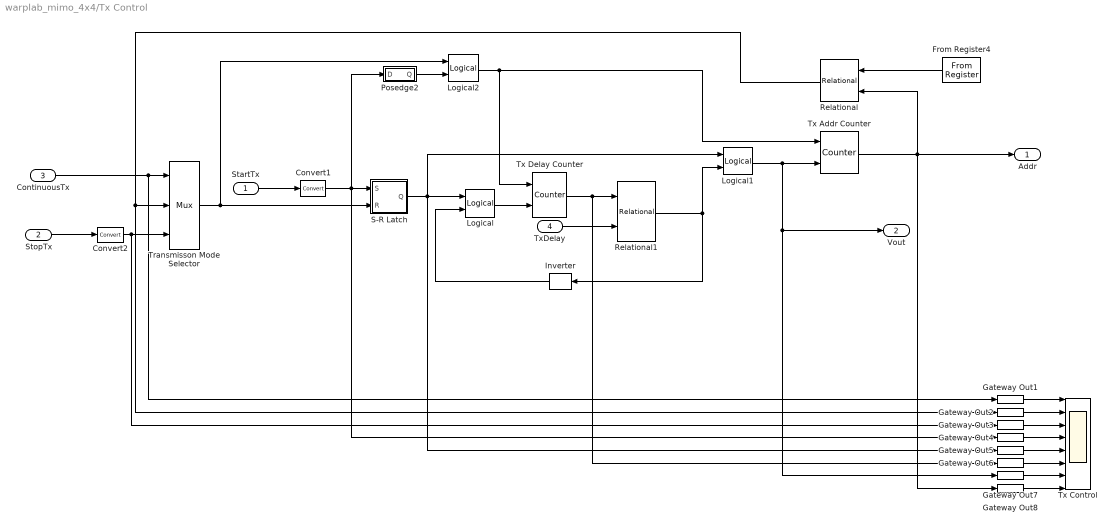
== system warplab_mimo_4x4/Tx Control ==
  StartTx : Inport
  StopTx : Inport  Port=2
  ContinuousTx : Inport  Port=3
  TxDelay : Inport  Port=4
  Convert1 : xbsIndex_r4/Convert  arith_type=Boolean  n_bits=1  bin_pt=0  quantization=Truncate  overflow=Wrap  latency=0  dbl_ovrd=off  pipeline=off  block_type=convert
  Convert2 : xbsIndex_r4/Convert  arith_type=Boolean  n_bits=1  bin_pt=0  quantization=Truncate  overflow=Wrap  latency=0  dbl_ovrd=off  pipeline=off  block_type=convert
  From Register4 : xbsIndex_r4/From Register  Orientation=left  shared_memory_name='TxLength'  init=2^14-1  period=1  ownership=Locally owned and initialized  arith_type=Unsigned  n_bits=14  bin_pt=0  dbl_ovrd=off  block_type=fromreg
      settings: AttributesFormatString=TxLength\n<< %<shared_memory_name> >>  infoedit="Register block that reads data to a shared memory register.  Delay of one sample period."  block_version=8.2
  Gateway Out{1..8} (8 alike) : xbsIndex_r4/Gateway Out  hdl_port=off  timing_constraint=None  locs_specified=off  LOCs={}  block_type=gatewayout
      settings: infoedit="Gateway out block.  Converts Xilinx fixed point inputs into ouputs of type Simulink integer, double, or fixed point.<P><P>Hardware notes:  In hardware these blocks become top level output ports or are discarded, depending on how they are configured."  block_version=10.1.2
  Inverter : xbsIndex_r4/Inverter  Orientation=left  en=off  latency=0  dbl_ovrd=off  block_type=inv
      settings: block_version=8.2
  Logical : xbsIndex_r4/Logical  logical_function=AND  inputs=2  en=off  latency=0  precision=Full  arith_type=Unsigned  n_bits=16  bin_pt=0  align_bp=on  dbl_ovrd=off  block_type=logical
      settings: block_version=8.2
  Logical1 : xbsIndex_r4/Logical  logical_function=AND  inputs=2  en=off  latency=0  precision=Full  arith_type=Unsigned  n_bits=16  bin_pt=0  align_bp=on  dbl_ovrd=off  block_type=logical
      settings: block_version=8.2
  Logical2 : xbsIndex_r4/Logical  logical_function=OR  inputs=2  en=off  latency=0  precision=Full  arith_type=Unsigned  n_bits=16  bin_pt=0  align_bp=on  dbl_ovrd=off  block_type=logical
      settings: block_version=8.2
  Posedge2 : Subsystem
  Relational : xbsIndex_r4/Relational  Orientation=left  mode=a<=b  en=off  latency=0  dbl_ovrd=off  block_type=relational
      settings: block_version=8.2
  Relational1 : xbsIndex_r4/Relational  mode=a>=b  en=off  latency=0  dbl_ovrd=off  block_type=relational
      settings: block_version=8.2
  S-R Latch : Subsystem
  Transmisson Mode Selector : xbsIndex_r4/Mux  inputs=2  en=off  latency=0  precision=Full  arith_type=Unsigned  n_bits=16  bin_pt=14  quantization=Truncate  overflow=Wrap  dbl_ovrd=off  block_type=mux
      settings: block_version=9.1.01
  Tx Addr Counter : xbsIndex_r4/Counter  cnt_type=Free Running  cnt_to=Inf  operation=Up  start_count=0  cnt_by_val=1  arith_type=Unsigned  n_bits=14  bin_pt=0  load_pin=off  rst=on  en=on  explicit_period=off  period=1  dbl_ovrd=off  use_behavioral_HDL=off  use_rpm=off  implementation=Fabric  block_type=counter
      settings: block_version=8.2
  Tx Control : Scope  NumInputPorts=8
      settings: TimeRange=70000  YMin=0~0~0~0~0~0~0~0  YMax=2~1~1~1~1~100~1~20000  SaveName=ScopeData3
  Tx Delay Counter : xbsIndex_r4/Counter  cnt_type=Free Running  cnt_to=Inf  operation=Up  start_count=0  cnt_by_val=1  arith_type=Unsigned  n_bits=14  bin_pt=0  load_pin=off  rst=on  en=on  explicit_period=off  period=1  dbl_ovrd=off  use_behavioral_HDL=off  use_rpm=off  implementation=Fabric  block_type=counter
      settings: block_version=8.2
  Addr : Outport
  Vout : Outport  Port=2
  wires:
  Transmisson Mode Selector/1 -> S-R Latch/2(R), Logical2/1
  Tx Delay Counter/1 -> Relational1/1, Gateway Out6/1
  TxDelay/1 -> Relational1/2
  ContinuousTx/1 -> Transmisson Mode Selector/1, Gateway Out1/1
  StartTx/1 -> Convert1/1
  StopTx/1 -> Convert2/1
  Logical/1 -> Tx Delay Counter/2
  S-R Latch/1(Q) -> Logical/1, Logical1/1, Gateway Out5/1
  Relational1/1 -> Inverter/1, Logical1/2
  Inverter/1 -> Logical/2
  Logical1/1 -> Tx Addr Counter/2, Vout/1, Gateway Out7/1
  Tx Addr Counter/1 -> Addr/1, Relational/2, Gateway Out8/1
  From Register4/1 -> Relational/1
  Posedge2/1(Q) -> Logical2/2
  Relational/1 -> Transmisson Mode Selector/2, Gateway Out2/1
  Logical2/1 -> Tx Addr Counter/1, Tx Delay Counter/1
  Convert1/1 -> S-R Latch/1(S), Posedge2/1(D), Gateway Out4/1
  Convert2/1 -> Transmisson Mode Selector/3, Gateway Out3/1
  Gateway Out5/1 -> Tx Control/5
  Gateway Out4/1 -> Tx Control/4
  Gateway Out3/1 -> Tx Control/3
  Gateway Out2/1 -> Tx Control/2
  Gateway Out1/1 -> Tx Control/1
  Gateway Out6/1 -> Tx Control/6
  Gateway Out7/1 -> Tx Control/7
  Gateway Out8/1 -> Tx Control/8

== system warplab_mimo_4x4/Radio 1 Rx Buffers/Radio 1 I/Q Buffer ==
  Addr_14b : Inport
  I/Q_32b : Inport  Port=2
  WE : Inport  Port=3
  Shared Memory : xbsIndex_r4/Shared Memory  shared_memory_name='RxBuff_Radio1'  depth=2^14  ownership=Locally Owned and Initialized  initVector=0  mutex=Unprotected  mode=Read and Write  write_mode=Read After Write  time_out=0  latency=1  explicit_data_type=on  arith_type=Unsigned  n_bits=32  bin_pt=0  implementation=Block RAM  use_rpm=off  block_type=shmem
      settings: AttributesFormatString=<< %<shared_memory_name> >>  block_version=10.1.2
  Terminator : Terminator
  wires:
  Addr_14b/1 -> Shared Memory/1
  I/Q_32b/1 -> Shared Memory/2
  WE/1 -> Shared Memory/3
  Shared Memory/1 -> Terminator/1
